simulink model "Induction_motor_modeling"  (R2016a)
settings: Solver=VariableStepAuto  StartTime=0.0  StopTime=2  MaxStep=1e-4  RelTol=1e-3
libraries: powerlib x10, powerlib_meascontrol x4
settings Model: Creator=AT Once  LastModifiedBy=AT Once

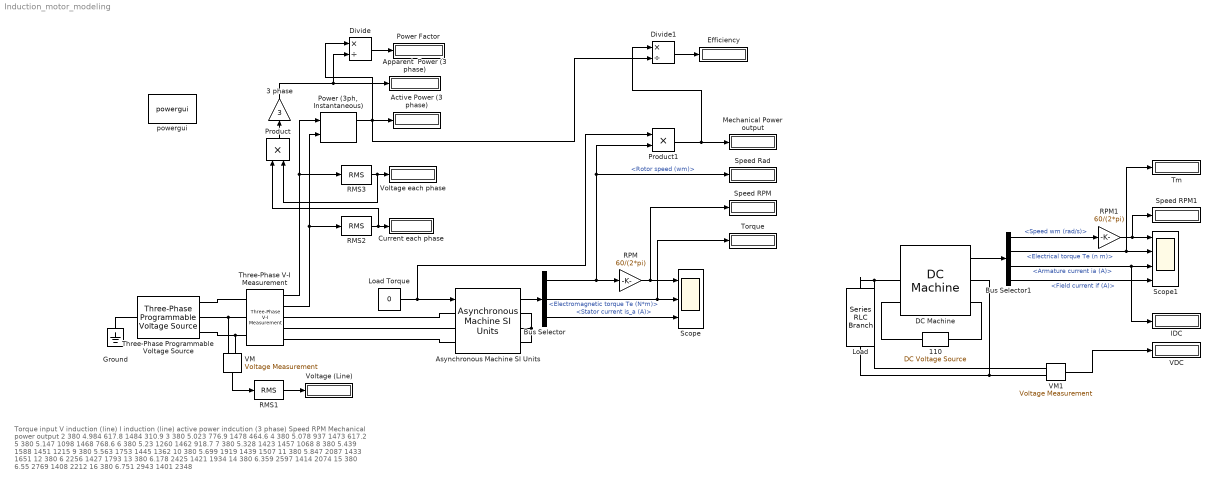
== system Induction_motor_modeling ==
  note: Torque input
      | V induction (line)
      | I induction (line)
      | active power indcution
      | (3 phase)
      | Speed RPM
      | Mechanical power output
      |
      | 2
      | 380
      | 4.984
      | 617.8
      | 1484
      | 310.9
      |
      | 3
      | 380
      | 5.023
      | 776.9
      | 1478
      | 464.6
      |
      | 4
      | 380
      | 5.078
      | 937
      | 1473
      | 617.2
      |
      | 5
      | 380
      | 5.147
      | 1098
      | 1468
      | 768.6
      |
      | 6
      | 380
      | 5.23
      | 1260
      | 1462
      | 918.7
      |
      | 7
      | 380
      | 5.328
      | 1423
      | 1457
      | 1068
      |
      | 8
      | 380
      | 5.439
      | 1588
      | 1451
      | 1215
      |
      | 9
      | 380
      | 5.563
      | 1753
      | 1445
      | 1362
      |
      | 10
      | 380
      | 5.699
      | 1919
      | 1439
      | 1507
      |
      | 11
      | 380
      | 5.847
      | 2087
      | 1433
      | 1651
      |
      | 12
      | 380
      | 6
      | 2256
      | 1427
      | 1793
      |
      | 13
      | 380
      | 6.178
      | 2425
      | 1421
      | 1934
      |
      | 14
      | 380
      | 6.359
      | 2597
      | 1414
      | 2074
      |
      | 15
      | 380
      | 6.55
      | 2769
      | 1408
      | 2212
      |
      | 16
      | 380
      | 6.751
      | 2943
      | 1401
      | 2348
  "110 " : powerlib/Electrical Sources/DC Voltage Source  Amplitude=110  Measurements=None
  3 phase : Gain  Gain=3
  Active Power (3 phase) : Display
  Apparent  Power (3 phase) : Display
  Asynchronous Machine SI Units : powerlib/Machines/Asynchronous Machine SI Units  RotorType=Wound  PresetModel=No  MechanicalLoad=Torque Tm  ShowDetailedParameters=on  ReferenceFrame=Stationary  Units=SI  MeasurementBus=off  NominalParameters=[2.2e+3 380 50]  Stator=[2.1484 9e-3]  Rotor=[2.831 9e-3]  Cage1=[0.4155 0.002066]  Cage2=[0.4168 0.0003495]  Lm=0.1318  Mechanical=[0.05 0.005879 2]  PolePairs=2  InitialConditions=[1 0 0 0 0 0 0 0]  SimulateSaturation=off  Saturation=[14.03593122, 27.81365428, 53.79336849, 72.68890987, 97.98006896, 148.6815601, 215.7428561, 302.9841135, 428.7778367 ; 230, 322, 414, 460, 506, 552, 598, 644, 690]  LoadFlowParameters=1492000  TsPowergui=0  TsBlock=-1  IterativeModel=Trapezoidal non iterative  IterativeDiscreteModel=Trapezoidal non iterative  Pmec=218.55
  Bus Selector : BusSelector  OutputSignals=Mechanical.Rotor speed (wm),Mechanical.Electromagnetic torque Te (N*m),Stator measurements.Stator current is_a (A)
  Bus Selector1 : BusSelector  OutputSignals=Speed wm (rad/s),Electrical torque Te (n m),Armature current ia (A),Field current if (A)
  Current each phase : Display
  DC Machine : powerlib/Machines/DC Machine  PresetModel=No  MechanicalLoad=Speed w  FieldType=Wound  ShowDetailedParameters=on  MeasurementBus=off  RLa="[ 1.45  0.012]"  RLf="[ 275  120]"  Laf=1.8  MachineConstant=Torque constant (N.m/A)  Ke=1.8  Kt=1.8  J=1  Bm=0  Tf=0  w0=0  Ifinit=0  TsPowergui=0  TsBlock=-1
  Divide : Product  Inputs=*/
  Divide1 : Product  Inputs=*/
  Efficiency : Display
  Ground : powerlib/Elements/Ground  LConnTagsString=a
  IDC : Display
  Load : powerlib/Elements/Series RLC Branch  LConnTagsString=__new0  RConnTagsString=__new0  BranchType=R  Resistance=100  Inductance=1e-3  SetiL0=off  InitialCurrent=0  Capacitance=1e-6  Setx0=off  InitialVoltage=0  Measurements=None
  Load Torque : Constant  Value=0
  Mechanical Power output : Display
  "Power (3ph, Instantaneous)" : powerlib_meascontrol/Measurements/Power (3ph, Instantaneous)
  Power Factor : Display
  Product : Product
  Product1 : Product
  RMS1 : powerlib_meascontrol/Measurements/RMS  TrueRMS=on  Freq=50  RMSInit=0  Ts=0
  RMS2 : powerlib_meascontrol/Measurements/RMS  TrueRMS=on  Freq=50  RMSInit=0  Ts=0
  RMS3 : powerlib_meascontrol/Measurements/RMS  TrueRMS=on  Freq=50  RMSInit=0  Ts=0
  RPM : Gain  Gain=60/(2*pi)
  RPM1 : Gain  Gain=60/(2*pi)
  Scope : Scope  NumInputPorts=3
  Scope1 : Scope  NumInputPorts=4
  Speed RPM : Display
  Speed RPM1 : Display
  Speed Rad : Display
  Three-Phase Programmable Voltage Source : powerlib/Electrical Sources/Three-Phase Programmable Voltage Source  PositiveSequence=[380 0 50]  VariationEntity=None  VariationType=Table of time-amplitude pairs  VariationTypeAlt=Step  VariationStep=0.5  VariationRate=10  VariationMagnitude=0.3  VariationFrequency=2  VariationTiming=[1 2]  VariationPhaseA=off  Amplitudes=[1 0.8 1.2 1.0]  TimeValues=[0 0.1 0.15 0.2]  HarmonicGeneration=off  HarmonicA=[3 0.2 -25 0]  HarmonicB=[2 0.15 35 2]  Timing="[0.05  3]"  BusType=swing  Pref=0  Qref=0  Qmin=-inf  Qmax=inf
  Three-Phase V-I Measurement : powerlib/Measurements/Three-Phase V-I Measurement  VoltageMeasurement=phase-to-ground  SetLabelV=off  LabelV=Vabc  Vpu=off  VpuLL=off  CurrentMeasurement=yes  SetLabelI=off  LabelI=Iabc  Ipu=off  Pbase=100e6  Vbase=500e3  OutputType=Complex  PhasorSimulation=off  PSBequivalent=0
  Tm : Display
  Torque : Display
  VDC : Display
  VM : powerlib/Measurements/Voltage Measurement  PhasorSimulation=off  OutputType=Complex  PSBequivalent=0
  VM1 : powerlib/Measurements/Voltage Measurement  PhasorSimulation=off  OutputType=Complex  PSBequivalent=0
  Voltage (Line) : Display
  Voltage each phase : Display
  powergui : powerlib/powergui  Priority=1  SimulationMode=Continuous  SolverType=Tustin/Backward Euler (TBE)  SampleTime=50e-6  frequency=60  SPID=off  DisableSnubberDevices=off  DisableRonSwitches=off  DisableVfSwitches=off  SwTol=0  DisplayEquations=off  Interpol=off  ExternalGateDelay=off  methode=off  Ts=10  FunctionMessages=off  echomessages=off  HookPort=off  EnableUseOfTLC=off  x0status=blocks  frequencyindice=0  Pbase=100e6  ErrMax=1e-4  Iterations=50  UnitsV=kV  UnitsW=MW  buscounter=0  RestoreLinks=warning  ResistiveCurrentMeasurement=off  Frange=[0:2:500]  Ylog=off  Xlog=on  ShowGrid=off  save=off  variable=ZData  structure=0  ZoomFFT=off  StartTime=0.0  cycles=1  DisplayStyle=1  fundamental=60  FreqAxis=off  MaxFrequency=1000  frequencyindicesteady=1  RmsSteady=1  display=off
  wires:
  RMS1/1 -> Voltage (Line)/1
  Asynchronous Machine SI Units/1 -> Bus Selector/1
  RMS2/1 -> Current each phase/1, Product/1
  RMS3/1 -> Voltage each phase/1, Product/2
  Bus Selector/1 -> Speed Rad/1, Product1/2, RPM/1  "<Rotor speed (wm)>"
  Bus Selector/2 -> Scope/2, Torque/1  "<Electromagnetic torque Te (N*m)>"
  RPM/1 -> Scope/1, Speed RPM/1
  Bus Selector/3 -> Scope/3  "<Stator current is_a (A)>"
  Divide/1 -> Power Factor/1
  Product1/1 -> Divide1/1, Mechanical Power output/1
  "Power (3ph, Instantaneous)"/1 -> Active Power (3 phase)/1, Divide1/2, Divide/1
  VM/1 -> RMS1/1
  Three-Phase V-I Measurement/1 -> "Power (3ph, Instantaneous)"/1, RMS3/1
  Three-Phase V-I Measurement/2 -> "Power (3ph, Instantaneous)"/2, RMS2/1
  Product/1 -> 3 phase/1
  DC Machine/1 -> Bus Selector1/1
  Bus Selector1/2 -> Scope1/2, Tm/1  "<Electrical torque Te (n m)>"
  Bus Selector1/3 -> IDC/1, Scope1/3  "<Armature current ia (A)>"
  Bus Selector1/4 -> Scope1/4  "<Field current if (A)>"
  VM1/1 -> VDC/1
  Bus Selector1/1 -> RPM1/1  "<Speed wm (rad/s)>"
  RPM1/1 -> Speed RPM1/1, Scope1/1
  3 phase/1 -> Divide/2, Apparent  Power (3 phase)/1
  Divide1/1 -> Efficiency/1
  Load Torque/1 -> Asynchronous Machine SI Units/1, Product1/1
  connections:
  Ground/LConn1 -- Three-Phase Programmable Voltage Source/LConn1
  Three-Phase Programmable Voltage Source/RConn2 -- VM/LConn2 -- Three-Phase V-I Measurement/LConn2
  Three-Phase V-I Measurement/LConn1 -- Three-Phase Programmable Voltage Source/RConn1
  Three-Phase V-I Measurement/LConn3 -- Three-Phase Programmable Voltage Source/RConn3 -- VM/LConn1
  Three-Phase V-I Measurement/RConn2 -- Asynchronous Machine SI Units/LConn2
  Three-Phase V-I Measurement/RConn1 -- Asynchronous Machine SI Units/LConn1
  "110 "/RConn1 -- DC Machine/LConn2
  "110 "/LConn1 -- DC Machine/RConn2
  VM1/LConn2 -- DC Machine/RConn1 -- Load/RConn1
  Three-Phase V-I Measurement/RConn3 -- Asynchronous Machine SI Units/LConn3
  Asynchronous Machine SI Units/RConn1 -- Asynchronous Machine SI Units/RConn2 -- Asynchronous Machine SI Units/RConn3
  Load/LConn1 -- DC Machine/LConn1 -- VM1/LConn1
